simulink model "fullQuad"  (R2015b)
settings: Solver=VariableStepAuto  StartTime=0.0  StopTime=10.0  RelTol=1e-3
undefined symbols (not defined in the file or in its folder): Kdz, Kiz, Kpz
settings Model: Creator=zammi  LastModifiedBy=zammi

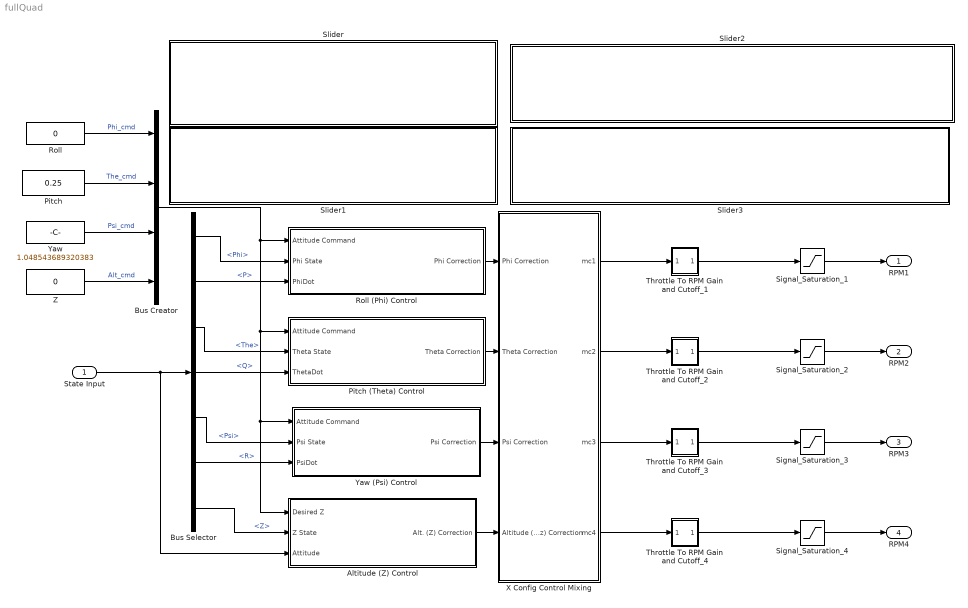
== system fullQuad ==
  State Input : Inport
  Altitude (Z) Control : Subsystem  mask{Kps=4, Kis=0.5, Kds=3.5, LimitOutput=on, USat=1, LSat=-1}
      mask prompts: Kps "Kp"; Kis "Ki"; Kds "Kd"; LimitOutput "Integral Saturation?"; USat "Upper saturation limit:"; LSat "Lower saturation limit:"
      mask help: Adjust PID controller gains through this mask interface, or "look under mask" for more detailed adjustments.
      mask TypeOptions Kps: Kps/Gain
      mask TypeOptions Kis: Kit/Gain
      mask TypeOptions Kds: Kds/Gain
      mask TypeOptions LimitOutput:
      | Integrator
      | Limited/LimitOutput
      mask TypeOptions USat:
      | Integrator
      | Limited/UpperSaturationLimit
      mask TypeOptions LSat:
      | Integrator
      | Limited/LowerSaturationLimit
      mask Display:
      | fprintf(['Kp = ' num2str(Kps) '\n' ...
      |     'Ki = ' num2str(Kis) '\n' ...
      |     'Kd = ' num2str(Kds) '\n' ...
      |     'Integral Saturation: ' LimitOutput]);
      | if strcmp(LimitOutput,'on')
      |     fprintf([' \n' ' \n' ' \n' ' \n' '\n' ...
      |         'Limits: ' num2str(USat) ' to ' num2str(LSat)]);
      | end
  Bus Creator : BusCreator  Inputs=4
  Bus Selector : BusSelector  OutputSignals=Phi,P,The,Q,Psi,R,Z
  Pitch : Constant  Value=0.25
  Pitch (Theta) Control : Subsystem  mask{Kpt=2, Kit=1.1, Kdt=1.2, LimitOutput=on, USat=1, LSat=-1}
      mask prompts: Kpt "Kp"; Kit "Ki"; Kdt "Kd"; LimitOutput "Integral Saturation?"; USat "Upper saturation limit:"; LSat "Lower saturation limit:"
      mask help: Adjust PID controller gains through this mask interface, or "look under mask" for more detailed adjustments.
      mask TypeOptions Kpt: Kpt/Gain
      mask TypeOptions Kit: Kit/Gain
      mask TypeOptions Kdt: Kdt/Gain
      mask TypeOptions LimitOutput:
      | Integrator
      | Limited/LimitOutput
      mask TypeOptions USat:
      | Integrator
      | Limited/UpperSaturationLimit
      mask TypeOptions LSat:
      | Integrator
      | Limited/LowerSaturationLimit
      mask Display:
      | fprintf(['Kp = ' num2str(Kpt) '\n' ...
      |     'Ki = ' num2str(Kit) '\n' ...
      |     'Kd = ' num2str(Kdt) '\n' ...
      |     'Integral Saturation: ' LimitOutput]);
      | if strcmp(LimitOutput,'on')
      |     fprintf([' \n' ' \n' ' \n' ' \n' '\n' ...
      |         'Limits: ' num2str(USat) ' to ' num2str(LSat)]);
      | end
  Roll : Constant  Value=0
  "Roll (Phi) Control " : Subsystem  mask{Kpp=2.0, Kip=1.1, Kdp=1.2, LimitOutput=on, USat=1, LSat=-1}
      mask prompts: Kpp "Kp"; Kip "Ki"; Kdp "Kd"; LimitOutput "Integral Saturation:"; USat "Upper saturation limit:"; LSat "Lower saturation limit:"
      mask help:
      | Adjust PID controller gains through this mask interface, or "look under mask"
      | for more detailed adjustments.
      mask TypeOptions Kpp: Kpp/Gain
      mask TypeOptions Kip: Kip/Gain
      mask TypeOptions Kdp: Kdp/Gain
      mask TypeOptions LimitOutput:
      | Integrator
      | Limited/LimitOutput
      mask TypeOptions USat:
      | Integrator
      | Limited/UpperSaturationLimit
      mask TypeOptions LSat:
      | Integrator
      | Limited/LowerSaturationLimit
      mask Display:
      | fprintf(['Kp = ' num2str(Kpp) '\n' ...
      |     'Ki = ' num2str(Kip) '\n' ...
      |     'Kd = ' num2str(Kdp) '\n'...
      |     'Integral Saturation: ' LimitOutput]);
      | if strcmp(LimitOutput,'on')
      |     fprintf([' \n' ' \n' ' \n' ' \n' '\n' ...
      |         'Limits: ' num2str(USat) ' to ' num2str(LSat)]);
      | end
  Signal_Saturation_{1..4} (4 alike) : Saturate  UpperLimit=100  LowerLimit=0
  Slider : Subsystem  DialogController=hmiCreateDDGDialog  IsWebBlock=on  mask(MWDashboardBlock){webBlockId=0419c70c-7b47-4291-9eac-865c63286a7b, webBlockType=slider, ShowInLibBrowser=on, ShowInitialText=on, HMISrcModelName=fullQuad}
      mask prompts: webBlockId "WebBlock Id"; webBlockType "WebBlock Type"; HMISrcModelName "Source Model"
      mask Help: helpview([docroot '/mapfiles/simulink.map'], 'hmi_slider')
      mask Display:
      | if strcmp(get_param(bdroot(gcb),'BlockDiagramType'), 'library')
      |     image([(matlabroot) '/toolbox/simulink/hmi/icons/Slider.png']);
      | end
  Slider1 : Subsystem  DialogController=hmiCreateDDGDialog  IsWebBlock=on  mask(MWDashboardBlock){webBlockId=4e81a138-6498-4852-bbd2-b98984e1b10d, webBlockType=slider, ShowInLibBrowser=on, ShowInitialText=on, HMISrcModelName=fullQuad}
      mask prompts: webBlockId "WebBlock Id"; webBlockType "WebBlock Type"; HMISrcModelName "Source Model"
      mask Help: helpview([docroot '/mapfiles/simulink.map'], 'hmi_slider')
      mask Display:
      | if strcmp(get_param(bdroot(gcb),'BlockDiagramType'), 'library')
      |     image([(matlabroot) '/toolbox/simulink/hmi/icons/Slider.png']);
      | end
  Slider2 : Subsystem  DialogController=hmiCreateDDGDialog  IsWebBlock=on  mask(MWDashboardBlock){webBlockId=8c4778a8-07db-4e45-b472-43a282c43db5, webBlockType=slider, ShowInLibBrowser=on, ShowInitialText=on, HMISrcModelName=fullQuad}
      mask prompts: webBlockId "WebBlock Id"; webBlockType "WebBlock Type"; HMISrcModelName "Source Model"
      mask Help: helpview([docroot '/mapfiles/simulink.map'], 'hmi_slider')
      mask Display:
      | if strcmp(get_param(bdroot(gcb),'BlockDiagramType'), 'library')
      |     image([(matlabroot) '/toolbox/simulink/hmi/icons/Slider.png']);
      | end
  Slider3 : Subsystem  DialogController=hmiCreateDDGDialog  IsWebBlock=on  mask(MWDashboardBlock){webBlockId=77a46dde-f482-42ed-a092-3b6eb75c3e55, webBlockType=slider, ShowInLibBrowser=on, ShowInitialText=on, HMISrcModelName=fullQuad}
      mask prompts: webBlockId "WebBlock Id"; webBlockType "WebBlock Type"; HMISrcModelName "Source Model"
      mask Help: helpview([docroot '/mapfiles/simulink.map'], 'hmi_slider')
      mask Display:
      | if strcmp(get_param(bdroot(gcb),'BlockDiagramType'), 'library')
      |     image([(matlabroot) '/toolbox/simulink/hmi/icons/Slider.png']);
      | end
  Throttle To RPM Gain and Cutoff_1 : Subsystem
  Throttle To RPM Gain and Cutoff_2 : Subsystem
  Throttle To RPM Gain and Cutoff_3 : Subsystem
  Throttle To RPM Gain and Cutoff_4 : Subsystem
  X Config Control Mixing : Subsystem
  Yaw : Constant  Value=1.048543689320383
  Yaw (Psi) Control : Subsystem  mask{Kps=4, Kis=0.5, Kds=3.5, LimitOutput=on, USat=1, LSat=-1}
      mask prompts: Kps "Kp"; Kis "Ki"; Kds "Kd"; LimitOutput "Integral Saturation?"; USat "Upper saturation limit:"; LSat "Lower saturation limit:"
      mask help: Adjust PID controller gains through this mask interface, or "look under mask" for more detailed adjustments.
      mask TypeOptions Kps: Kps/Gain
      mask TypeOptions Kis: Kit/Gain
      mask TypeOptions Kds: Kds/Gain
      mask TypeOptions LimitOutput:
      | Integrator
      | Limited/LimitOutput
      mask TypeOptions USat:
      | Integrator
      | Limited/UpperSaturationLimit
      mask TypeOptions LSat:
      | Integrator
      | Limited/LowerSaturationLimit
      mask Display:
      | fprintf(['Kp = ' num2str(Kps) '\n' ...
      |     'Ki = ' num2str(Kis) '\n' ...
      |     'Kd = ' num2str(Kds) '\n' ...
      |     'Integral Saturation: ' LimitOutput]);
      | if strcmp(LimitOutput,'on')
      |     fprintf([' \n' ' \n' ' \n' ' \n' '\n' ...
      |         'Limits: ' num2str(USat) ' to ' num2str(LSat)]);
      | end
  Z : Constant  Value=0
  RPM1 : Outport
  RPM2 : Outport  Port=2
  RPM3 : Outport  Port=3
  RPM4 : Outport  Port=4
  wires:
  Z/1 -> Bus Creator/4  "Alt_cmd"
  Yaw/1 -> Bus Creator/3  "Psi_cmd"
  Pitch/1 -> Bus Creator/2  "The_cmd"
  Roll/1 -> Bus Creator/1  "Phi_cmd"
  Bus Selector/6 -> Yaw (Psi) Control/3(PsiDot)  "<R>"
  Bus Selector/4 -> Pitch (Theta) Control/3(ThetaDot)  "<Q>"
  Bus Selector/2 -> "Roll (Phi) Control "/3(PhiDot)  "<P>"
  Bus Selector/3 -> Pitch (Theta) Control/2(Theta State)  "<The>"
  Bus Selector/7 -> Altitude (Z) Control/2(Z State)  "<Z>"
  Bus Selector/5 -> Yaw (Psi) Control/2(Psi State)  "<Psi>"
  State Input/1 -> Altitude (Z) Control/3(Attitude), Bus Selector/1
  Bus Selector/1 -> "Roll (Phi) Control "/2(Phi State)  "<Phi>"
  "Roll (Phi) Control "/1(Phi Correction) -> X Config Control Mixing/1(Phi Correction)
  Pitch (Theta) Control/1(Theta Correction) -> X Config Control Mixing/2(Theta Correction)
  Altitude (Z) Control/1(Alt. (Z) Correction) -> X Config Control Mixing/4(Altitude (z) Correction)
  Yaw (Psi) Control/1(Psi Correction) -> X Config Control Mixing/3(Psi Correction)
  Throttle To RPM Gain and Cutoff_4/1(Out5) -> Signal_Saturation_4/1
  Throttle To RPM Gain and Cutoff_3/1(Out5) -> Signal_Saturation_3/1
  Throttle To RPM Gain and Cutoff_2/1(Out) -> Signal_Saturation_2/1
  Throttle To RPM Gain and Cutoff_1/1(Out5) -> Signal_Saturation_1/1
  X Config Control Mixing/4(mc4) -> Throttle To RPM Gain and Cutoff_4/1(In5)
  X Config Control Mixing/3(mc3) -> Throttle To RPM Gain and Cutoff_3/1(In5)
  X Config Control Mixing/2(mc2) -> Throttle To RPM Gain and Cutoff_2/1(In)
  X Config Control Mixing/1(mc1) -> Throttle To RPM Gain and Cutoff_1/1(In5)
  Signal_Saturation_1/1 -> RPM1/1
  Signal_Saturation_2/1 -> RPM2/1
  Signal_Saturation_4/1 -> RPM4/1
  Signal_Saturation_3/1 -> RPM3/1
  Bus Creator/1 -> Altitude (Z) Control/1(Desired Z), Yaw (Psi) Control/1(Attitude Command), Pitch (Theta) Control/1(Attitude Command), "Roll (Phi) Control "/1("Attitude Command ")

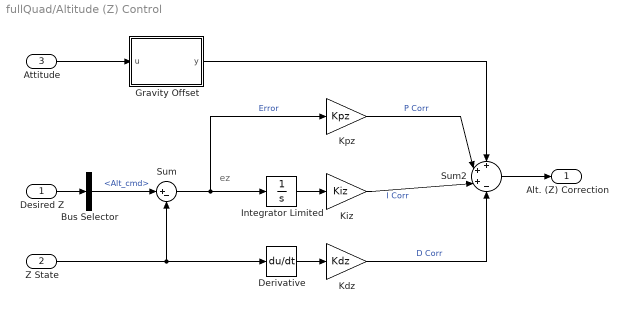
== system fullQuad/Altitude (Z) Control ==
  note: ez
  Desired Z : Inport
  Z State : Inport  Port=2
  Attitude : Inport  Port=3
  Bus Selector : BusSelector  OutputSignals=Alt_cmd
  Derivative : Derivative
  Gravity Offset : MATLAB Function  TreatAsAtomicUnit=on
  Integrator Limited : Integrator  LimitOutput=on  UpperSaturationLimit=USat  LowerSaturationLimit=LSat
  Kdz : Gain  Gain=Kdz
  Kiz : Gain  Gain=Kiz
  Kpz : Gain  Gain=Kpz
  Sum : Sum  Inputs=|+-
  Sum2 : Sum  Inputs=+++-
  Alt. (Z) Correction : Outport
  wires:
  Gravity Offset/1(y) -> Sum2/1
  Desired Z/1 -> Bus Selector/1
  Z State/1 -> Derivative/1, Sum/2
  Sum2/1 -> Alt. (Z) Correction/1
  Kpz/1 -> Sum2/2  "P Corr"
  Sum/1 -> Integrator Limited/1, Kpz/1  "Error"
  Kiz/1 -> Sum2/3  "I Corr"
  Kdz/1 -> Sum2/4  "D Corr"
  Integrator Limited/1 -> Kiz/1
  Bus Selector/1 -> Sum/1  "<Alt_cmd>"
  Derivative/1 -> Kdz/1
  Attitude/1 -> Gravity Offset/1(u)

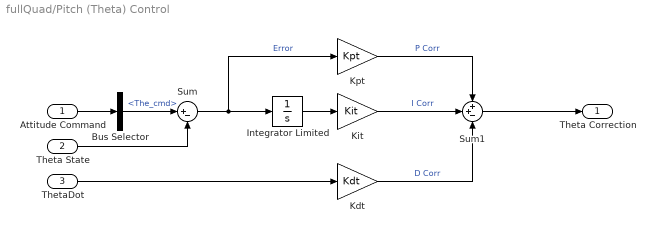
== system fullQuad/Pitch (Theta) Control ==
  Attitude Command : Inport
  Theta State : Inport  Port=2
  ThetaDot : Inport  Port=3
  Bus Selector : BusSelector  OutputSignals=The_cmd
  Integrator Limited : Integrator  LimitOutput=on  UpperSaturationLimit=USat  LowerSaturationLimit=LSat
  Kdt : Gain  Gain=Kdt
  Kit : Gain  Gain=Kit
  Kpt : Gain  Gain=Kpt
  Sum : Sum  Inputs=|+-
  Sum1 : Sum  Inputs=++-
  Theta Correction : Outport
  wires:
  Sum/1 -> Integrator Limited/1, Kpt/1  "Error"
  Attitude Command/1 -> Bus Selector/1
  Theta State/1 -> Sum/2
  Sum1/1 -> Theta Correction/1
  Kpt/1 -> Sum1/1  "P Corr"
  Kdt/1 -> Sum1/3  "D Corr"
  Kit/1 -> Sum1/2  "I Corr"
  Integrator Limited/1 -> Kit/1
  Bus Selector/1 -> Sum/1  "<The_cmd>"
  ThetaDot/1 -> Kdt/1

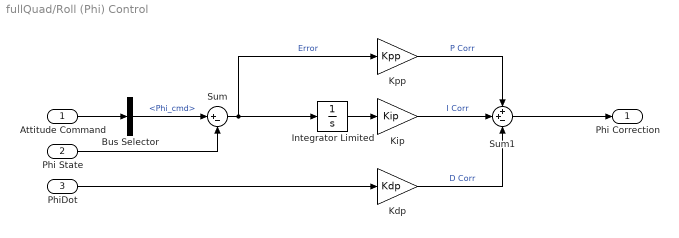
== system fullQuad/Roll (Phi) Control  ==
  "Attitude Command " : Inport
  Phi State : Inport  Port=2
  PhiDot : Inport  Port=3
  Bus Selector : BusSelector  OutputSignals=Phi_cmd
  Integrator Limited : Integrator  LimitOutput=on  UpperSaturationLimit=USat  LowerSaturationLimit=LSat
  Kdp : Gain  Gain=Kdp
  Kip : Gain  Gain=Kip
  Kpp : Gain  Gain=Kpp
  Sum : Sum  Inputs=|+-
  Sum1 : Sum  Inputs=++-
  Phi Correction : Outport
  wires:
  Sum/1 -> Integrator Limited/1, Kpp/1  "Error"
  Phi State/1 -> Sum/2
  Sum1/1 -> Phi Correction/1
  Kpp/1 -> Sum1/1  "P Corr"
  Kdp/1 -> Sum1/3  "D Corr"
  Kip/1 -> Sum1/2  "I Corr"
  Integrator Limited/1 -> Kip/1
  "Attitude Command "/1 -> Bus Selector/1
  Bus Selector/1 -> Sum/1  "<Phi_cmd>"
  PhiDot/1 -> Kdp/1

== system fullQuad/Slider ==

== system fullQuad/Slider1 ==

== system fullQuad/Slider2 ==

== system fullQuad/Slider3 ==

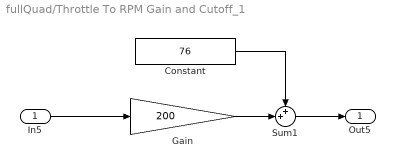
== system fullQuad/Throttle To RPM Gain and Cutoff_1 ==
  In5 : Inport
  Constant : Constant  Value=76
  Gain : Gain  Gain=200
  Sum1 : Sum  Inputs=++|
  Out5 : Outport
  wires:
  Sum1/1 -> Out5/1
  In5/1 -> Gain/1
  Gain/1 -> Sum1/2
  Constant/1 -> Sum1/1

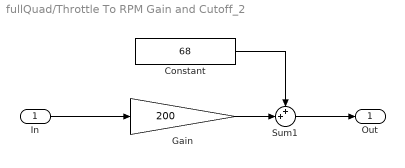
== system fullQuad/Throttle To RPM Gain and Cutoff_2 ==
  In : Inport
  Constant : Constant  Value=68
  Gain : Gain  Gain=200
  Sum1 : Sum  Inputs=++|
  Out : Outport
  wires:
  Sum1/1 -> Out/1
  In/1 -> Gain/1
  Gain/1 -> Sum1/2
  Constant/1 -> Sum1/1

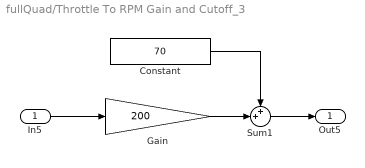
== system fullQuad/Throttle To RPM Gain and Cutoff_3 ==
  In5 : Inport
  Constant : Constant  Value=70
  Gain : Gain  Gain=200
  Sum1 : Sum  Inputs=++|
  Out5 : Outport
  wires:
  Sum1/1 -> Out5/1
  In5/1 -> Gain/1
  Gain/1 -> Sum1/2
  Constant/1 -> Sum1/1

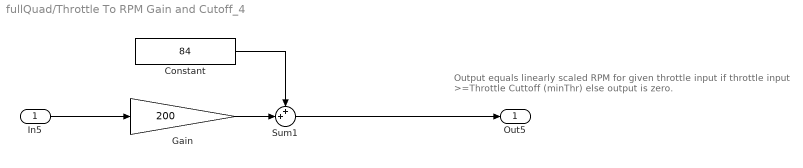
== system fullQuad/Throttle To RPM Gain and Cutoff_4 ==
  note: Output equals linearly scaled RPM
      | for given throttle input if throttle input >=Throttle Cuttoff (minThr)
      | else output is zero.
  In5 : Inport
  Constant : Constant  Value=84
  Gain : Gain  Gain=200
  Sum1 : Sum  Inputs=++|
  Out5 : Outport
  wires:
  Sum1/1 -> Out5/1
  In5/1 -> Gain/1
  Gain/1 -> Sum1/2
  Constant/1 -> Sum1/1

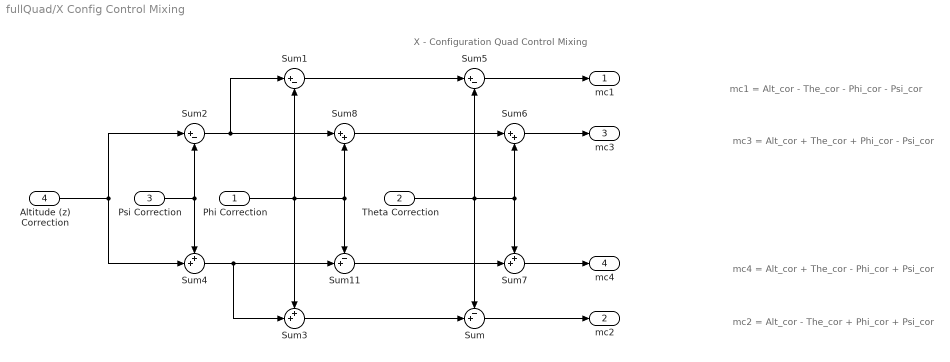
== system fullQuad/X Config Control Mixing ==
  note: mc1 = Alt_cor - The_cor - Phi_cor - Psi_cor
  note: X - Configuration Quad Control Mixing
  note: mc3 = Alt_cor + The_cor + Phi_cor - Psi_cor
  note: mc2 = Alt_cor - The_cor + Phi_cor + Psi_cor
  note: mc4 = Alt_cor + The_cor - Phi_cor + Psi_cor
  Phi Correction : Inport
  Theta Correction : Inport  Port=2
  Psi Correction : Inport  Port=3
  Altitude (z) Correction : Inport  Port=4
  Sum : Sum  Inputs=-+|
  Sum1 : Sum  Inputs=|+-
  Sum11 : Sum  Inputs=-+|
  Sum2 : Sum  Inputs=|+-
  Sum3 : Sum  Inputs=++|
  Sum4 : Sum  Inputs=++|
  Sum5 : Sum  Inputs=|+-
  Sum6 : Sum  Inputs=|++
  Sum7 : Sum  Inputs=++|
  Sum8 : Sum  Inputs=|++
  mc1 : Outport
  mc2 : Outport  Port=2
  mc3 : Outport  Port=3
  mc4 : Outport  Port=4
  wires:
  Sum2/1 -> Sum8/1, Sum1/1
  Psi Correction/1 -> Sum4/1, Sum2/2
  Phi Correction/1 -> Sum3/1, Sum1/2, Sum8/2, Sum11/1
  Sum4/1 -> Sum3/2, Sum11/2
  Sum3/1 -> Sum/2
  Theta Correction/1 -> Sum7/1, Sum6/2, Sum5/2, Sum/1
  Sum1/1 -> Sum5/1
  Sum8/1 -> Sum6/1
  Sum11/1 -> Sum7/2
  Sum5/1 -> mc1/1
  Sum6/1 -> mc3/1
  Sum7/1 -> mc4/1
  Altitude (z) Correction/1 -> Sum2/1, Sum4/2
  Sum/1 -> mc2/1

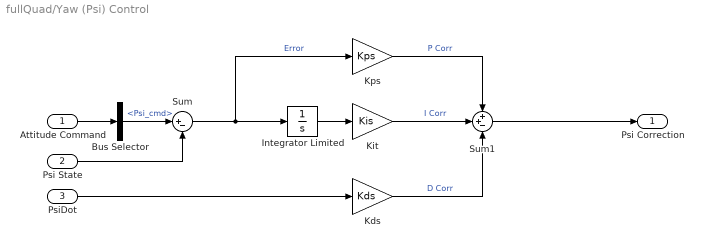
== system fullQuad/Yaw (Psi) Control ==
  Attitude Command : Inport
  Psi State : Inport  Port=2
  PsiDot : Inport  Port=3
  Bus Selector : BusSelector  OutputSignals=Psi_cmd
  Integrator Limited : Integrator  LimitOutput=on  UpperSaturationLimit=USat  LowerSaturationLimit=LSat
  Kds : Gain  Gain=Kds
  Kit : Gain  Gain=Kis
  Kps : Gain  Gain=Kps
  Sum : Sum  Inputs=|+-
  Sum1 : Sum  Inputs=++-
  Psi Correction : Outport
  wires:
  Sum/1 -> Integrator Limited/1, Kps/1  "Error"
  Attitude Command/1 -> Bus Selector/1
  Sum1/1 -> Psi Correction/1
  Psi State/1 -> Sum/2
  Kps/1 -> Sum1/1  "P Corr"
  Kds/1 -> Sum1/3  "D Corr"
  Kit/1 -> Sum1/2  "I Corr"
  Integrator Limited/1 -> Kit/1
  Bus Selector/1 -> Sum/1  "<Psi_cmd>"
  PsiDot/1 -> Kds/1

== matlab function fullQuad/Altitude (Z) Control/Gravity Offset ==
  data: u input; y output
function y = fcn(u)
%#codegen
c1 = cosd(YPR(1));c2 = cosd(YPR(2));c3 = cosd(YPR(3));
s1 = sind(YPR(1));s2 = sind(YPR(2));s3 = sind(YPR(3));
DCM =  [c2*c1 c2*s1 -s2;...
        s3*s2*c1-c3*s1 s3*s2*s1+c3*c1 s3*c2;...
        c3*s2*c1+s3*s1 c3*s2*s1-s3*c1 c3*c2];


y = u;
